simulink model "QPSK_Rayleigh_differential_coding"  (R2019b)
settings: Solver=VariableStepAuto  StartTime=0.0  StopTime=1  RelTol=1e-3
undefined symbols (not defined in the file or in its folder): doppler
libraries: commchan3 x2, commutil2 x2, commdigbbndpm3 x2, commrandsrc3 x1, commsink2 x1
settings Model: Creator=Nikhil  LastModifiedBy=Nikhil

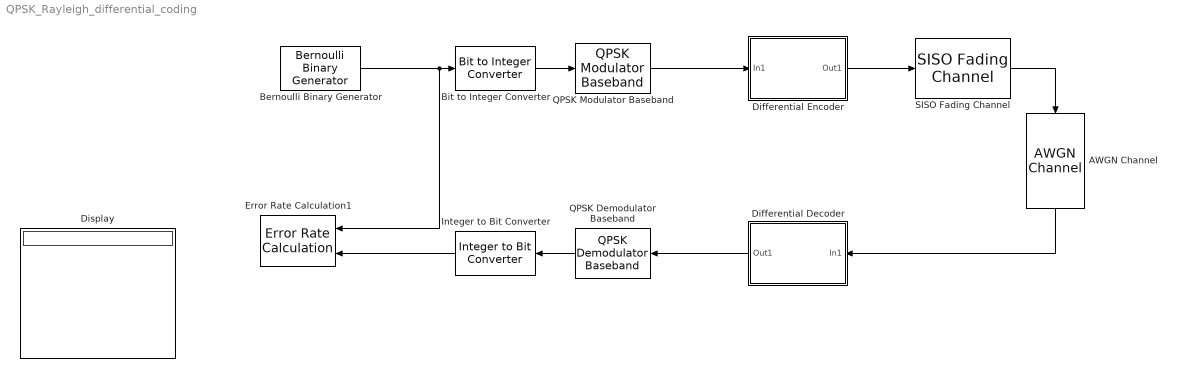
== system QPSK_Rayleigh_differential_coding ==
  AWGN Channel : commchan3/AWGN Channel  InputProcessing=Columns as channels (frame based)  seed=117  noiseMode="Signal to noise ratio  (SNR)"  EbNodB=10  EsNodB=10  SNRdB=s  bitsPerSym=1  Ps=1  Tsym=1  variance=1
      settings: SourceProductName=Communications Toolbox
  Bernoulli Binary Generator : commrandsrc3/Bernoulli Binary Generator  ProbabilityOfZero=0.5  SeedSource=Auto  Seed=322  SampleTime=1e-6  SamplesPerFrame=2  OutputDataType=uint8  SimulateUsing=Interpreted execution
      settings: SourceProductName=Communications Toolbox
  Bit to Integer Converter : commutil2/Bit to Integer Converter  nbits=2  bitOrder=MSB first  signedOutputValues=Unsigned  outDtype=Inherit via internal rule  outDtypeSigned=Inherit via internal rule
      settings: SourceProductName=Communications Toolbox
  Differential Decoder : Subsystem
  Differential Encoder : Subsystem
  Display : Display
  Error Rate Calculation1 : commsink2/Error Rate Calculation  N=0  st_delay=0  cp_mode=Entire frame  subframe=[]  PMode=Workspace  WsName=ErrorVec  RsMode2=off  stop=off  numErr=100  maxBits=1e6
      settings: SourceProductName=Communications Toolbox
  Integer to Bit Converter : commutil2/Integer to Bit Converter  nbits=2  signedInputValues=Unsigned  bitOrder=MSB first  outDtype=Inherit via internal rule
      settings: SourceProductName=Communications Toolbox
  QPSK Demodulator Baseband : commdigbbndpm3/QPSK Demodulator Baseband  OutType=Integer  DecType=Hard decision  VarSource=Dialog  Variance=1  Dec=Gray  Ph=pi/4  outDtype1=Inherit via internal rule  outDtype2=Inherit via internal rule  derotateFactorWordLen=16  derotateFactorDataTypeStr=Inherit: Same word length as input  derotateFactorLastDataTypeStr=Inherit: Same word length as input
      settings: SourceProductName=Communications Toolbox
  QPSK Modulator Baseband : commdigbbndpm3/QPSK Modulator Baseband  InType=Integer  Enc=Gray  Ph=pi/4  outDtype=Inherit via back propagation  outWordLen=16  outUDDataType=sfix(16)  outFracLenMode=Best precision  outFracLen=15  outDataTypeStr=Inherit: Inherit via back propagation  outLastDataTypeStr=Inherit: Inherit via back propagation
      settings: SourceProductName=Communications Toolbox
  SISO Fading Channel : commchan3/SISO Fading Channel  InheritSampleRate=on  SampleRate=1  PathDelays=[0, 1.8e-5]  AveragePathGains=[0,3]  NormalizePathGains=on  FadingDistribution=Rayleigh  KFactor=3  DirectPathDopplerShift=0  DirectPathInitialPhase=0  MaximumDopplerShift=100  DopplerSpectrum=doppler('Flat')  RandomStream=mt19937ar with seed  Seed=77  PathGainsOutputPort=off  ChannelFilterDelayOutputPort=off  SimulateUsing=Interpreted execution  Visualization=Off  PathsForDopplerDisplay=1  SamplesToDisplay=25%
      settings: SourceProductName=Communications Toolbox
  wires:
  Bit to Integer Converter/1 -> QPSK Modulator Baseband/1
  Integer to Bit Converter/1 -> Error Rate Calculation1/2
  QPSK Demodulator Baseband/1 -> Integer to Bit Converter/1
  Differential Decoder/1(Out1) -> QPSK Demodulator Baseband/1
  Bernoulli Binary Generator/1 -> Error Rate Calculation1/1, Bit to Integer Converter/1
  QPSK Modulator Baseband/1 -> Differential Encoder/1(In1)
  Differential Encoder/1(Out1) -> SISO Fading Channel/1
  SISO Fading Channel/1 -> AWGN Channel/1
  AWGN Channel/1 -> Differential Decoder/1(In1)

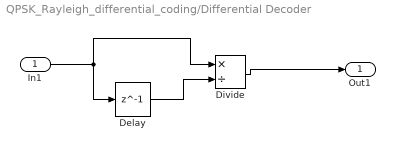
== system QPSK_Rayleigh_differential_coding/Differential Decoder ==
  In1 : Inport
  Delay : Delay  DelayLength=1  InitialCondition=1
  Divide : Product  Inputs=*/
  Out1 : Outport
  wires:
  In1/1 -> Delay/1, Divide/1
  Divide/1 -> Out1/1
  Delay/1 -> Divide/2

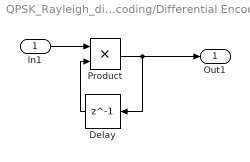
== system QPSK_Rayleigh_differential_coding/Differential Encoder ==
  In1 : Inport
  Delay : Delay  DelayLength=1  InitialCondition=1
  Product : Product
  Out1 : Outport
  wires:
  In1/1 -> Product/1
  Product/1 -> Delay/1, Out1/1
  Delay/1 -> Product/2
